simulink model "tau_9"  (R2019b)
settings: Solver=VariableStepAuto  StartTime=0.0  StopTime=100  RelTol=1e-3
libraries: simulink x2
settings Model: Creator=Sergey  LastModifiedBy=Sergey

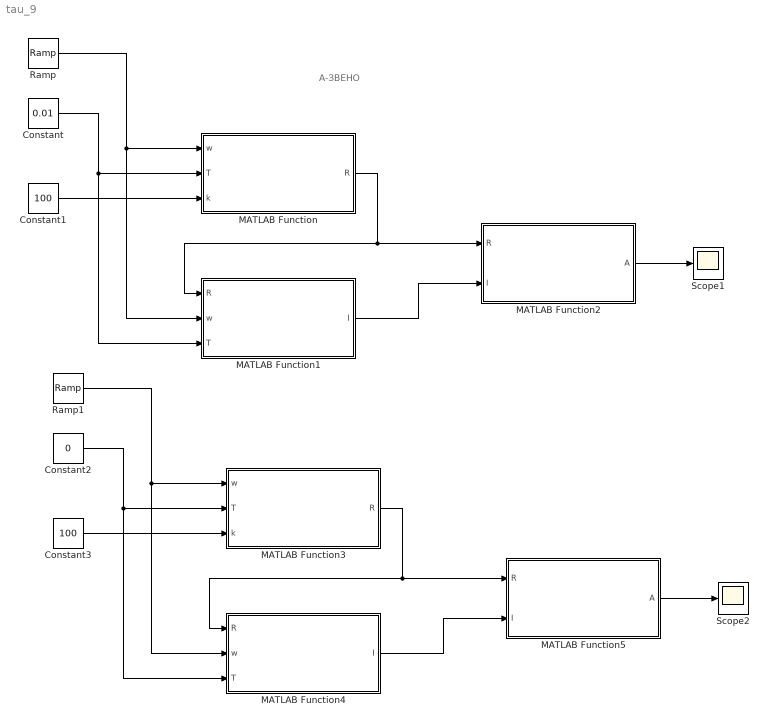
== system tau_9 ==
  note: А-ЗВЕНО
  Constant : Constant  Value=0.01
  Constant1 : Constant  Value=100
  Constant2 : Constant  Value=0
  Constant3 : Constant  Value=100
  MATLAB Function : MATLAB Function  TreatAsAtomicUnit=on
  MATLAB Function1 : MATLAB Function  TreatAsAtomicUnit=on
  MATLAB Function2 : MATLAB Function  TreatAsAtomicUnit=on
  MATLAB Function3 : MATLAB Function  TreatAsAtomicUnit=on
  MATLAB Function4 : MATLAB Function  TreatAsAtomicUnit=on
  MATLAB Function5 : MATLAB Function  TreatAsAtomicUnit=on
  Ramp : simulink/Sources/Ramp  slope=1  start=0  InitialOutput=0
  Ramp1 : simulink/Sources/Ramp  slope=1  start=0  InitialOutput=0
  Scope1 : Scope
  Scope2 : Scope
  wires:
  Ramp/1 -> MATLAB Function1/2(w), MATLAB Function/1(w)
  Constant/1 -> MATLAB Function1/3(T), MATLAB Function/2(T)
  Constant1/1 -> MATLAB Function/3(k)
  MATLAB Function/1(R) -> MATLAB Function1/1(R), MATLAB Function2/1(R)
  MATLAB Function1/1(I) -> MATLAB Function2/2(I)
  MATLAB Function2/1(A) -> Scope1/1
  MATLAB Function5/1(A) -> Scope2/1
  MATLAB Function4/1(I) -> MATLAB Function5/2(I)
  MATLAB Function3/1(R) -> MATLAB Function5/1(R), MATLAB Function4/1(R)
  Constant3/1 -> MATLAB Function3/3(k)
  Constant2/1 -> MATLAB Function3/2(T), MATLAB Function4/3(T)
  Ramp1/1 -> MATLAB Function3/1(w), MATLAB Function4/2(w)

== matlab function tau_9/MATLAB Function1 ==
  data: R input; w input; I output; T input
function I = fcn(R,w,T)

I = R*w*T;
I = -I;

== matlab function tau_9/MATLAB Function ==
  data: w input; R output; T input; k input
function R = fcn(w,T,k)

R = k/(1+w^2*T^2);

== matlab function tau_9/MATLAB Function2 ==
  data: R input; I input; A output
function A = fcn(R,I)

A = R^2+I^2;
A = sqrt(A);

== matlab function tau_9/MATLAB Function3 ==
  data: w input; R output; T input; k input
function R = fcn(w,T,k)

R = k/(1+w^2*T^2);

== matlab function tau_9/MATLAB Function4 ==
  data: R input; w input; I output; T input
function I = fcn(R,w,T)

I = R*w*T;
I = -I;

== matlab function tau_9/MATLAB Function5 ==
  data: R input; I input; A output
function A = fcn(R,I)

A = R^2+I^2;
A = sqrt(A);
